simulink model "Pruebas_ag2pos"  (R2022b)
settings: Solver=VariableStepAuto  StartTime=0.0  StopTime=0.01  RelTol=1e-3
libraries: simulink x5
settings Model: Creator=emate  LastModifiedBy=USUARIO

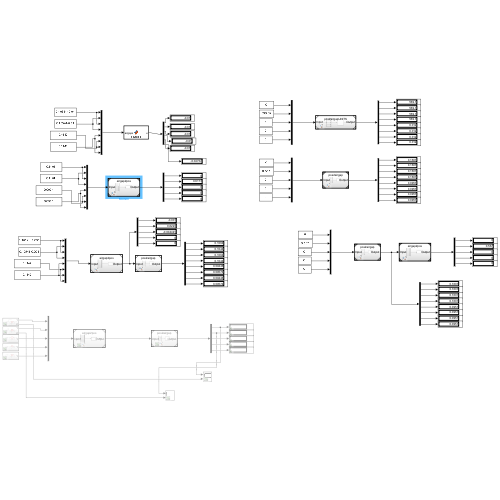
[thumbnail: Simulink's stored preview of the top-level diagram]
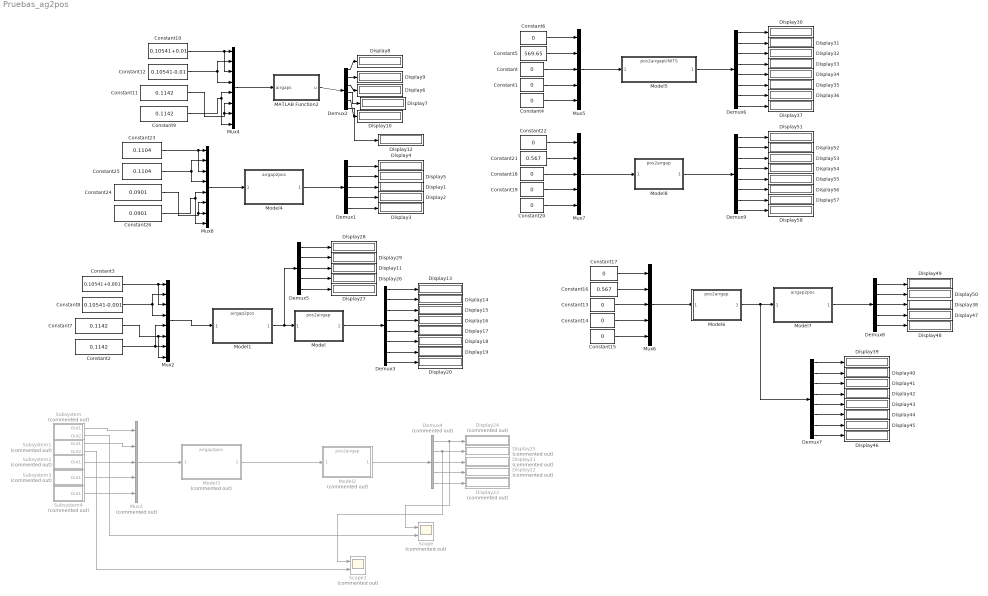
== system Pruebas_ag2pos ==
  Constant{,1,4,6,13..15,17..20,22} (12 alike) : Constant  Value=0
  Constant10 : Constant  Value=0.10541+0.01
  Constant{2,7,9,11} (4 alike) : Constant  Value=0.1142
  Constant12 : Constant  Value=0.10541-0.01
  Constant16 : Constant  Value=0.567
  Constant21 : Constant  Value=0.567
  Constant23 : Constant  Value=0.1104
  Constant24 : Constant  Value=0.0901
  Constant25 : Constant  Value=0.1104
  Constant26 : Constant  Value=0.0901
  Constant3 : Constant  Value=0.10541+0.001
  Constant5 : Constant  Value=569.65
  Constant8 : Constant  Value=0.10541-0.001
  Demux1 : Demux  Outputs=5
  Demux2 : Demux  Outputs=6
  Demux{3,6..7,9} (4 alike) : Demux  Outputs=8
  Demux4 : Demux  Commented=on  Outputs=5
  Demux5 : Demux  Outputs=5
  Demux8 : Demux  Outputs=5
  Display{1..20,26..58} (53 alike) : Display
  Display{21..25} (5 alike) : Display  Commented=on
  MATLAB Function2 : MATLAB Function  TreatAsAtomicUnit=on
  Model : ModelReference  ModelNameDialog=pos2airgap.slx  SimulationMode=Normal  ModelReferenceVersion=1.7
  Model1 : ModelReference  ModelNameDialog=airgap2pos.slx  SimulationMode=Normal  ModelReferenceVersion=1.8
  Model2 : ModelReference  Commented=on  ModelNameDialog=pos2airgap.slx  SimulationMode=Normal  ModelReferenceVersion=1.7
  Model3 : ModelReference  Commented=on  ModelNameDialog=airgap2pos.slx  SimulationMode=Normal  ModelReferenceVersion=1.8
  Model4 : ModelReference  ModelNameDialog=airgap2pos.slx  SimulationMode=Normal  ModelReferenceVersion=1.8
  Model5 : ModelReference  ModelNameDialog=pos2airgapUNITS.slx  SimulationMode=Normal  ModelReferenceVersion=1.3
  Model6 : ModelReference  ModelNameDialog=pos2airgap.slx  SimulationMode=Normal  ModelReferenceVersion=1.7
  Model7 : ModelReference  ModelNameDialog=airgap2pos.slx  SimulationMode=Normal  ModelReferenceVersion=1.8
  Model8 : ModelReference  ModelNameDialog=pos2airgap.slx  SimulationMode=Normal  ModelReferenceVersion=1.7
  Mux2 : Mux  Inputs=8
  Mux3 : Mux  Commented=on  Inputs=5
  Mux4 : Mux  Inputs=8
  Mux5 : Mux  Inputs=5
  Mux6 : Mux  Inputs=5
  Mux7 : Mux  Inputs=5
  Mux8 : Mux  Inputs=8
  Scope : Scope  Commented=on  NumInputPorts=2
  Scope1 : Scope  Commented=on  NumInputPorts=2
  Subsystem : Subsystem  Commented=on
  Subsystem1 : Subsystem  Commented=on
  Subsystem2 : Subsystem  Commented=on
  Subsystem3 : Subsystem  Commented=on
  Subsystem4 : Subsystem  Commented=on
  wires:
  Mux2/1 -> Model1/1
  Demux3/5 -> Display17/1
  Demux3/6 -> Display18/1
  Demux3/1 -> Display13/1
  Demux3/2 -> Display14/1
  Demux3/8 -> Display20/1
  Demux3/7 -> Display19/1
  Model/1 -> Demux3/1
  Demux3/4 -> Display16/1
  Demux3/3 -> Display15/1
  Subsystem4/1(Out1) -> Mux3/5
  Subsystem/1(Out1) -> Mux3/1
  Subsystem2/1(Out1) -> Mux3/3
  Subsystem3/1(Out1) -> Mux3/4
  Subsystem1/1(Out1) -> Mux3/2
  Mux3/1 -> Model3/1
  Model2/1 -> Demux4/1
  Demux4/3 -> Display21/1
  Demux4/2 -> Scope1/1, Display25/1
  Demux4/4 -> Display22/1
  Demux4/1 -> Scope/1, Display24/1
  Demux4/5 -> Display23/1
  Demux1/5 -> Display3/1
  Demux1/4 -> Display2/1
  Demux1/3 -> Display1/1
  Demux1/2 -> Display5/1
  Model4/1 -> Demux1/1
  Demux1/1 -> Display4/1
  MATLAB Function2/1(u) -> Demux2/1
  Demux2/1 -> Display8/1
  Demux2/2 -> Display9/1
  Demux2/3 -> Display6/1
  Demux2/4 -> Display7/1
  Constant9/1 -> Mux4/8, Mux4/5
  Mux4/1 -> MATLAB Function2/1(airgaps)
  Constant10/1 -> Mux4/3, Mux4/1
  Constant12/1 -> Mux4/2, Mux4/4
  Constant11/1 -> Mux4/6, Mux4/7
  Demux2/5 -> Display10/1
  Demux2/6 -> Display12/1
  Constant2/1 -> Mux2/7, Mux2/5
  Constant3/1 -> Mux2/3, Mux2/1
  Constant8/1 -> Mux2/2, Mux2/4
  Constant7/1 -> Mux2/8, Mux2/6
  Demux5/2 -> Display29/1
  Demux5/1 -> Display28/1
  Demux5/3 -> Display11/1
  Demux5/4 -> Display26/1
  Demux5/5 -> Display27/1
  Model1/1 -> Demux5/1, Model/1
  Demux6/5 -> Display34/1
  Demux6/1 -> Display30/1
  Demux6/4 -> Display33/1
  Demux6/6 -> Display35/1
  Demux6/7 -> Display36/1
  Model5/1 -> Demux6/1
  Demux6/8 -> Display37/1
  Demux6/3 -> Display32/1
  Demux6/2 -> Display31/1
  Mux5/1 -> Model5/1
  Constant/1 -> Mux5/3
  Constant4/1 -> Mux5/5
  Constant1/1 -> Mux5/4
  Constant5/1 -> Mux5/2
  Constant6/1 -> Mux5/1
  Subsystem/2(Out2) -> Scope/2
  Subsystem1/2(Out2) -> Scope1/2
  Model3/1 -> Model2/1
  Demux8/1 -> Display49/1
  Demux8/4 -> Display47/1
  Demux8/2 -> Display50/1
  Model7/1 -> Demux8/1
  Demux8/3 -> Display38/1
  Demux8/5 -> Display48/1
  Constant17/1 -> Mux6/1
  Constant16/1 -> Mux6/2
  Constant14/1 -> Mux6/4
  Constant13/1 -> Mux6/3
  Constant15/1 -> Mux6/5
  Mux6/1 -> Model6/1
  Model6/1 -> Demux7/1, Model7/1
  Demux7/2 -> Display40/1
  Demux7/5 -> Display43/1
  Demux7/8 -> Display46/1
  Demux7/4 -> Display42/1
  Demux7/6 -> Display44/1
  Demux7/3 -> Display41/1
  Demux7/1 -> Display39/1
  Demux7/7 -> Display45/1
  Demux9/3 -> Display53/1
  Constant20/1 -> Mux7/5
  Constant21/1 -> Mux7/2
  Demux9/6 -> Display56/1
  Demux9/5 -> Display55/1
  Constant22/1 -> Mux7/1
  Constant19/1 -> Mux7/4
  Mux7/1 -> Model8/1
  Model8/1 -> Demux9/1
  Demux9/8 -> Display58/1
  Demux9/2 -> Display52/1
  Demux9/7 -> Display57/1
  Demux9/1 -> Display51/1
  Constant18/1 -> Mux7/3
  Demux9/4 -> Display54/1
  Mux8/1 -> Model4/1
  Constant24/1 -> Mux8/6, Mux8/7
  Constant23/1 -> Mux8/3, Mux8/1
  Constant25/1 -> Mux8/2, Mux8/4
  Constant26/1 -> Mux8/8, Mux8/5

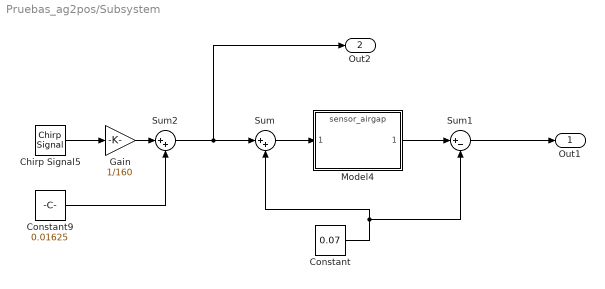
== system Pruebas_ag2pos/Subsystem ==
  Chirp Signal5 : simulink/Sources/Chirp Signal  f1=0.1  T=4  f2=1
  Constant : Constant  Value=0.07
  Constant9 : Constant  Value=0.01625
  Gain : Gain  Gain=1/160
  Model4 : ModelReference  ModelNameDialog=sensor_airgap.slx  SimulationMode=Normal  ModelReferenceVersion=1.3
  Sum : Sum  Inputs=|++
  Sum1 : Sum  Inputs=|+-
  Sum2 : Sum  Inputs=|++
  Out1 : Outport
  Out2 : Outport  Port=2
  wires:
  Sum/1 -> Model4/1
  Constant/1 -> Sum1/2, Sum/2
  Chirp Signal5/1 -> Gain/1
  Sum1/1 -> Out1/1
  Constant9/1 -> Sum2/2
  Model4/1 -> Sum1/1
  Gain/1 -> Sum2/1
  Sum2/1 -> Out2/1, Sum/1

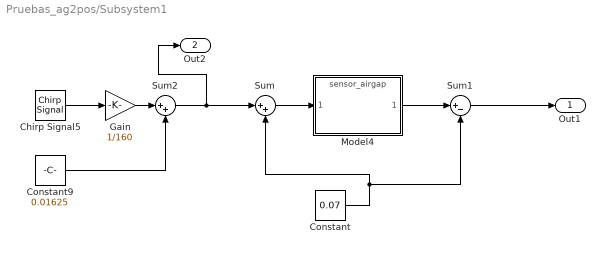
== system Pruebas_ag2pos/Subsystem1 ==
  Chirp Signal5 : simulink/Sources/Chirp Signal  f1=0.1  T=4  f2=1
  Constant : Constant  Value=0.07
  Constant9 : Constant  Value=0.01625
  Gain : Gain  Gain=1/160
  Model4 : ModelReference  ModelNameDialog=sensor_airgap.slx  SimulationMode=Normal  ModelReferenceVersion=1.3
  Sum : Sum  Inputs=|++
  Sum1 : Sum  Inputs=|+-
  Sum2 : Sum  Inputs=|++
  Out1 : Outport
  Out2 : Outport  Port=2
  wires:
  Sum/1 -> Model4/1
  Constant/1 -> Sum1/2, Sum/2
  Chirp Signal5/1 -> Gain/1
  Sum1/1 -> Out1/1
  Constant9/1 -> Sum2/2
  Model4/1 -> Sum1/1
  Gain/1 -> Sum2/1
  Sum2/1 -> Out2/1, Sum/1

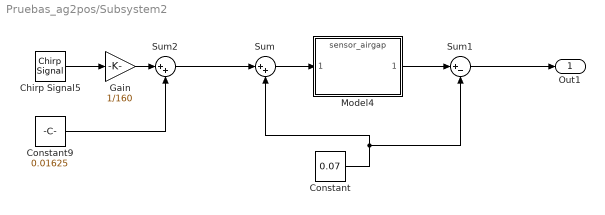
== system Pruebas_ag2pos/Subsystem2 ==
  Chirp Signal5 : simulink/Sources/Chirp Signal  f1=0.1  T=4  f2=1
  Constant : Constant  Value=0.07
  Constant9 : Constant  Value=0.01625
  Gain : Gain  Gain=1/160
  Model4 : ModelReference  ModelNameDialog=sensor_airgap.slx  SimulationMode=Normal  ModelReferenceVersion=1.3
  Sum : Sum  Inputs=|++
  Sum1 : Sum  Inputs=|+-
  Sum2 : Sum  Inputs=|++
  Out1 : Outport
  wires:
  Sum/1 -> Model4/1
  Constant/1 -> Sum1/2, Sum/2
  Chirp Signal5/1 -> Gain/1
  Sum1/1 -> Out1/1
  Constant9/1 -> Sum2/2
  Model4/1 -> Sum1/1
  Gain/1 -> Sum2/1
  Sum2/1 -> Sum/1

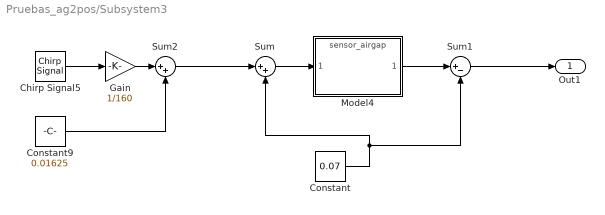
== system Pruebas_ag2pos/Subsystem3 ==
  Chirp Signal5 : simulink/Sources/Chirp Signal  f1=0.1  T=4  f2=1
  Constant : Constant  Value=0.07
  Constant9 : Constant  Value=0.01625
  Gain : Gain  Gain=1/160
  Model4 : ModelReference  ModelNameDialog=sensor_airgap.slx  SimulationMode=Normal  ModelReferenceVersion=1.3
  Sum : Sum  Inputs=|++
  Sum1 : Sum  Inputs=|+-
  Sum2 : Sum  Inputs=|++
  Out1 : Outport
  wires:
  Sum/1 -> Model4/1
  Constant/1 -> Sum1/2, Sum/2
  Chirp Signal5/1 -> Gain/1
  Sum1/1 -> Out1/1
  Constant9/1 -> Sum2/2
  Model4/1 -> Sum1/1
  Gain/1 -> Sum2/1
  Sum2/1 -> Sum/1

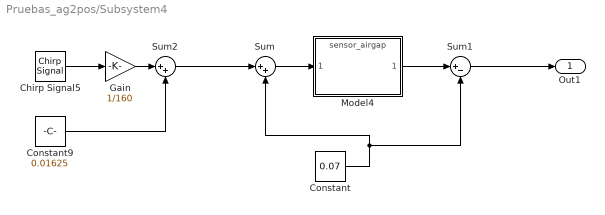
== system Pruebas_ag2pos/Subsystem4 ==
  Chirp Signal5 : simulink/Sources/Chirp Signal  f1=0.1  T=4  f2=1
  Constant : Constant  Value=0.07
  Constant9 : Constant  Value=0.01625
  Gain : Gain  Gain=1/160
  Model4 : ModelReference  ModelNameDialog=sensor_airgap.slx  SimulationMode=Normal  ModelReferenceVersion=1.3
  Sum : Sum  Inputs=|++
  Sum1 : Sum  Inputs=|+-
  Sum2 : Sum  Inputs=|++
  Out1 : Outport
  wires:
  Sum/1 -> Model4/1
  Constant/1 -> Sum1/2, Sum/2
  Chirp Signal5/1 -> Gain/1
  Sum1/1 -> Out1/1
  Constant9/1 -> Sum2/2
  Model4/1 -> Sum1/1
  Gain/1 -> Sum2/1
  Sum2/1 -> Sum/1

== matlab function Pruebas_ag2pos/MATLAB Function2 ==
  data: airgaps input; u output
function u = ag2pos(airgaps)

% CONSTANTES

x_sragy = 0.8069; 
y_sragy = 0.1142;
z_sragy = 0.10825; 

x_sragz = 0.81231;
y_sragz = 0.2114;
z_sragz = -0.0396; 

z_infr = 0.6328;

coder.varsize('rotx_aux');
coder.varsize('roty_aux');
coder.varsize('rotz_aux');
coder.varsize('y_aux');
coder.varsize('z_aux');

rotx_aux=zeros(2,1);
roty_aux=zeros(2,1);
rotz_aux=zeros(2,1);
y_aux=zeros(4,1);
z_aux=zeros(4,1);

% ROTACIONES
rotx_aux(1) = asin((airgaps(2) - airgaps(1))/(2*y_sragz));
rotx_aux(2) = asin((airgaps(4) - airgaps(3))/(2*y_sragz));

roty_aux(1) = asin((airgaps(1) - airgaps(3))/(2*x_sragz));
roty_aux(2) = asin((airgaps(2) - airgaps(4))/(2*x_sragz));

rotz_aux(1) = asin((airgaps(5) - airgaps(7))/(2*x_sragy));
rotz_aux(2) = asin((airgaps(8) - airgaps(6))/(2*x_sragy));

rotx = mean(rotx_aux);
roty = mean(roty_aux);
rotz = mean(rotz_aux);

% DISTANCIAS
y_aux(1) = + airgaps(5) - y_sragy * cos(rotz) - x_sragy * sin(rotz) + y_sragz * sin(rotx);
y_aux(2) = - airgaps(6) + y_sragy * cos(rotz) - x_sragy * sin(rotz) + y_sragz * sin(rotx);
y_aux(3) = + airgaps(7) - y_sragy * cos(rotz) + x_sragy * sin(rotz) + y_sragz * sin(rotx);
y_aux(4) = - airgaps(8) + y_sragy * cos(rotz) + x_sragy * sin(rotz) + y_sragz * sin(rotx);

z_aux(1) = z_infr - airgaps(1) - z_sragz * cos(roty) + x_sragz * sin(roty) - y_sragz * sin(rotx);
z_aux(2) = z_infr - airgaps(2) - z_sragz * cos(roty) + x_sragz * sin(roty) + y_sragz * sin(rotx);
z_aux(3) = z_infr - airgaps(3) - z_sragz * cos(roty) - x_sragz * sin(roty) - y_sragz * sin(rotx);
z_aux(4) = z_infr - airgaps(4) - z_sragz * cos(roty) - x_sragz * sin(roty) + y_sragz * sin(rotx);


y = mean(y_aux);

u =[y_aux(1),y_aux(2),y_aux(3),y_aux(4),y, rotx]';
